simulink model "DCDC3_CL"  (R2024a)
settings: Solver=VariableStepAuto  StartTime=0.0  StopTime=Tsim_outLoop  FixedStep=Tstep  RelTol=1e-3
values from neighbouring files (symbols this model uses):
  deadtimesw = 2.8e-6    (= 2.8e-06)    [DCDC_param.m]
  ILmax = 3    [DCDC_param.m]
  Rload = VoutNom/IoutNom    (= 39.6825396825)    [DCDC_param.m]
  Tsw = 2.8e-6    (= 2.8e-06)    [DCDC_param.m]
  VinNom = 30    [DCDC_param.m]
  VoutNom = 50    [DCDC_param.m]
undefined symbols (not defined in the file or in its folder): den_aaf, DiscIntNeverNeededParam, kaw_i, kaw_v, ki_i, ki_v, kp_i, kp_v, kpf_i, kpf_v, num_aaf, Tstep, VLlim, zden_pf_i, zden_pf_v, znum_pf_i, znum_pf_v
libraries: simulink x30, nesl_utility x20, fl_lib x19, spsTriangleGeneratorLib x18, ee_lib x7
(part 1 of 2)
settings Model: Creator=nicholas  LastModifiedBy=nicholas
settings RTWCC: GPUComputeCapability=3.5

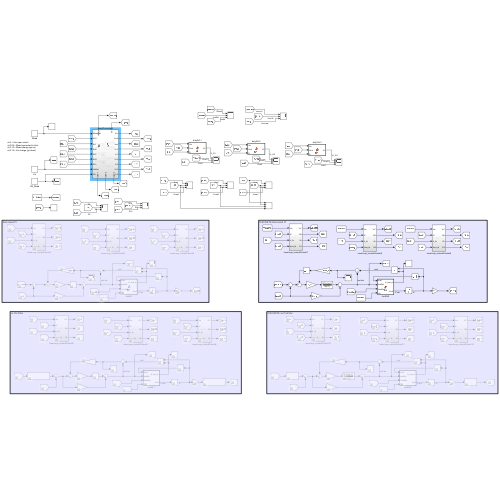
[thumbnail: Simulink's stored preview of the top-level diagram]
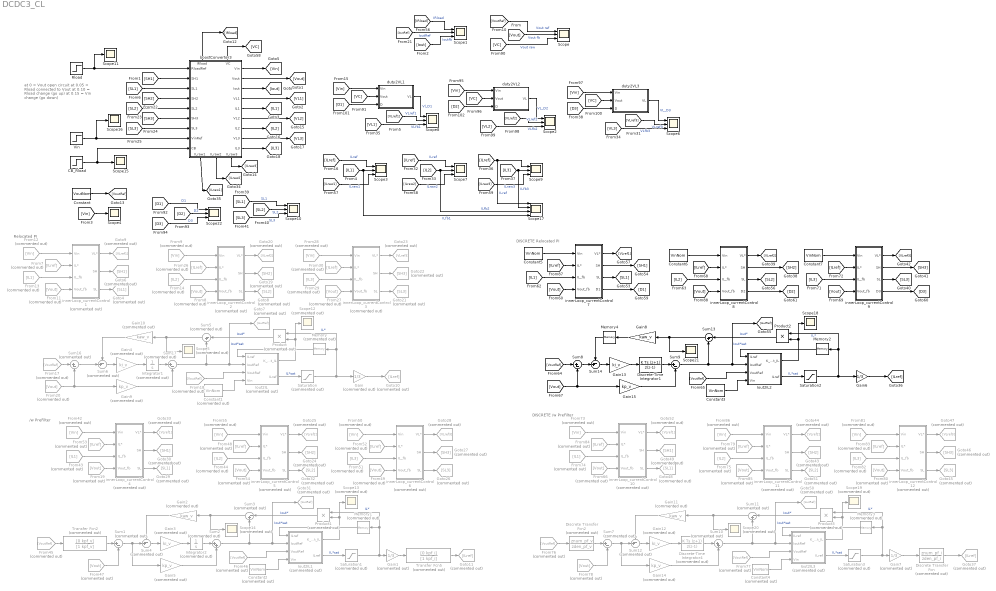
== system DCDC3_CL ==
  note: Relocated PI
  note: /w PreFilter
  note: at 0 = Vout open circuit
      | at 0.05 = Rload connected to Vout
      | at 0.10 = Rload change (go up)
      | at 0.15 = Vin change (go down)
  note: DISCRETE Relocated PI
  note: DISCRETE /w PreFilter
  CB_Rload : Step  Time=0.05  SampleTime=0
  Constant : Constant  Value=VoutNom
  Constant1 : Constant  Commented=on  Value=VinNom
  Constant2 : Constant  Commented=on  Value=VinNom
  Constant{3,5..7} (4 alike) : Constant  Value=VinNom
  Constant4 : Constant  Commented=on  Value=VinNom
  Discrete Transfer Fcn : DiscreteTransferFcn  Commented=on  Numerator=znum_pf_i  Denominator=zden_pf_i
  Discrete Transfer Fcn2 : DiscreteTransferFcn  Commented=on  Numerator=znum_pf_v  Denominator=zden_pf_v
  Discrete-Time Integrator1 : DiscreteIntegrator  IntegratorMethod=Integration: Trapezoidal  SampleTime=Tsw  ICPrevOutput=DiscIntNeverNeededParam  ICPrevScaledInput=DiscIntNeverNeededParam
  Discrete-Time Integrator4 : DiscreteIntegrator  Commented=on  IntegratorMethod=Integration: Trapezoidal  SampleTime=Tsw  ICPrevOutput=DiscIntNeverNeededParam  ICPrevScaledInput=DiscIntNeverNeededParam
  From{8,11,19..20,27,47,49,54,66,78,80,85} (12 alike) : From  Commented=on  GotoTag=Vout
  From{9,12,28,42,50,55,73,81,86} (9 alike) : From  Commented=on  GotoTag=Vin
  From13 : From  Commented=on  GotoTag=IL1
  From14 : From  Commented=on  GotoTag=IL2
  From{17..18,45..46,76..77} (6 alike) : From  Commented=on  GotoTag=VoutRef
  From{7,26,30,48,52..53,79,83..84} (9 alike) : From  Commented=on  GotoTag=ILref
  From29 : From  Commented=on  GotoTag=IL3
  From43 : From  Commented=on  GotoTag=IL1
  From44 : From  Commented=on  GotoTag=IL2
  From51 : From  Commented=on  GotoTag=IL3
  From74 : From  Commented=on  GotoTag=IL1
  From75 : From  Commented=on  GotoTag=IL2
  From82 : From  Commented=on  GotoTag=IL3
  Gain : Gain  Commented=on  Gain=1/3
  Gain1 : Gain  Commented=on  Gain=1/3
  Gain10 : Gain  Commented=on  Gain=kaw_v
  Gain11 : Gain  Commented=on  Gain=kaw_v
  Gain12 : Gain  Commented=on  Gain=ki_v
  Gain13 : Gain  Gain=ki_v
  Gain14 : Gain  Commented=on  Gain=kp_v
  Gain15 : Gain  Gain=kp_v
  Gain2 : Gain  Commented=on  Gain=kaw_v
  Gain3 : Gain  Commented=on  Gain=ki_v
  Gain4 : Gain  Commented=on  Gain=ki_v
  Gain5 : Gain  Commented=on  Gain=kp_v
  Gain6 : Gain  Gain=1/3
  Gain7 : Gain  Commented=on  Gain=1/3
  Gain8 : Gain  Gain=kaw_v
  Gain9 : Gain  Commented=on  Gain=kp_v
  Goto10 : Goto  Commented=on  GotoTag=ILref
  Goto11 : Goto  Commented=on  GotoTag=ILref
  Goto19 : Goto  Commented=on  GotoTag=SH2
  Goto20 : Goto  Commented=on  GotoTag=VLref2
  Goto21 : Goto  Commented=on  GotoTag=SL3
  Goto22 : Goto  Commented=on  GotoTag=SH3
  Goto23 : Goto  Commented=on  GotoTag=VLref3
  Goto24 : Goto  Commented=on  GotoTag=SH2
  Goto25 : Goto  Commented=on  GotoTag=VLref2
  Goto26 : Goto  Commented=on  GotoTag=SL3
  Goto27 : Goto  Commented=on  GotoTag=SH3
  Goto28 : Goto  Commented=on  GotoTag=VLref3
  Goto29 : Goto  Commented=on  GotoTag=SL1
  Goto30 : Goto  Commented=on  GotoTag=SH1
  Goto31 : Goto  Commented=on  GotoTag=IoutRef
  Goto32 : Goto  Commented=on  GotoTag=SL2
  Goto33 : Goto  Commented=on  GotoTag=VLref1
  Goto37 : Goto  Commented=on  GotoTag=ILref
  Goto4 : Goto  Commented=on  GotoTag=SL1
  Goto43 : Goto  Commented=on  GotoTag=SH2
  Goto44 : Goto  Commented=on  GotoTag=VLref2
  Goto45 : Goto  Commented=on  GotoTag=SL3
  Goto46 : Goto  Commented=on  GotoTag=SH3
  Goto47 : Goto  Commented=on  GotoTag=VLref3
  Goto48 : Goto  Commented=on  GotoTag=SL1
  Goto49 : Goto  Commented=on  GotoTag=SH1
  Goto50 : Goto  Commented=on  GotoTag=IoutRef
  Goto51 : Goto  Commented=on  GotoTag=SL2
  Goto52 : Goto  Commented=on  GotoTag=VLref1
  Goto6 : Goto  Commented=on  GotoTag=SH1
  Goto7 : Goto  Commented=on  GotoTag=IoutRef
  Goto8 : Goto  Commented=on  GotoTag=SL2
  Goto9 : Goto  Commented=on  GotoTag=VLref1
  Integrator1 : Integrator  Commented=on
  Integrator2 : Integrator  Commented=on
  Iout2IL : MATLAB Function  Commented=on  TreatAsAtomicUnit=on
  Iout2IL1 : MATLAB Function  Commented=on  TreatAsAtomicUnit=on
  Iout2IL2 : MATLAB Function  TreatAsAtomicUnit=on
  Iout2IL3 : MATLAB Function  Commented=on  TreatAsAtomicUnit=on
  Memory : Memory  Commented=on
  Memory1 : Memory  Commented=on
  Memory2 : Memory
  Memory3 : Memory  Commented=on
  Memory4 : Memory
  Product : Product  Commented=on
  Product1 : Product  Commented=on
  Product2 : Product
  Product3 : Product  Commented=on
  Rload : Step  Time=0.1  Before=Rload  After=Rload*2  SampleTime=0
  Saturation : Saturate  Commented=on  UpperLimit=ILmax  LowerLimit=-ILmax
  Saturation1 : Saturate  Commented=on  UpperLimit=ILmax  LowerLimit=-ILmax
  Saturation2 : Saturate  UpperLimit=ILmax  LowerLimit=-ILmax
  Saturation3 : Saturate  Commented=on  UpperLimit=ILmax  LowerLimit=-ILmax
  Scope{,1..3,6..10,22} (10 alike) : Scope  NumInputPorts=3
  Scope{4,11,15..16,18,21} (6 alike) : Scope
  Scope{5,12..14,19..20} (6 alike) : Scope  Commented=on
  Scope17 : Scope  NumInputPorts=4
  Sum{1,7,16..17} (4 alike) : Sum  Commented=on  Inputs=|+-
  Sum10 : Sum  Commented=on  Inputs=|++
  Sum11 : Sum  Commented=on  Inputs=|-+
  Sum12 : Sum  Commented=on  Inputs=-+|
  Sum13 : Sum  Inputs=|-+
  Sum14 : Sum  Inputs=-+|
  Sum2 : Sum  Commented=on  Inputs=|++
  Sum3 : Sum  Commented=on  Inputs=|-+
  Sum4 : Sum  Commented=on  Inputs=-+|
  Sum5 : Sum  Commented=on  Inputs=|-+
  Sum6 : Sum  Commented=on  Inputs=-+|
  Sum8 : Sum  Inputs=|+-
  Sum9 : Sum  Inputs=|+-
  Transfer Fcn2 : TransferFcn  Commented=on  Numerator=[0 kpf_v]  Denominator=[1 kpf_v]
  Transfer Fcn5 : TransferFcn  Commented=on  Numerator=[0 kpf_i]  Denominator=[1 kpf_i]
  Vin : Step  Time=0.15  Before=VinNom  After=20  SampleTime=0
  boostConverter3 : Subsystem
      settings: PortSchema="{\"entries\":[{\"content\":{\"sides\":[{\"content\":{\"connectorIds\":[\"In1\",\"In2\",\"In3\",\"In4\",\"In5\",\"In6\",\"In7\",\"In8\",\"In9\"]},\"type\":\"ConnectorPlacement.EquallySpacedRectSide\",\"uuid\":\"b55511d0-facb-4a91-89ed-441d6ed333ad\"},{\"content\":{\"connectorIds\":[\"Out1\",\"Out2\",\"Out3\",\"Out4\",\"Out5\",\"Out6\",\"Out7\",\"Out8\",\"Out9\"],\"side\":\"RIGHT\"},\"type\":\"ConnectorPlacement.EquallySpacedRectSide\",\"uuid\":\"ead4c989-543f-44ce-a846-94a06a8e7cad\"},{\"content\":{\"connectorIds\":[\"Out13\",\"Out14\"],\"side\":\"TOP\"},\"type\":\"ConnectorPlacement.EquallySpacedRectSide\",\"uuid\":\"5dda5bdb-be03-4339-a562-891a6c50bbdd\"},{\"content\":{\"connectorIds\":[\"Out10\",\"Out11\",\"Out12\"],\"side\":\"BOTTOM\"},\"type\":\"ConnectorPlacement.EquallySpacedRectSide\",\"uuid\":\"6ce891dd-de23-45e8-b9d4-5962e703d661\"}]},\"type\":\"ConnectorPlacement.EquallySpacedConnector\",\"uuid\":\"250b2e18-3b96-4cfc-be30-976dd92f9027\"}],\"packageUris\":[\"http://schema.mathworks.com/mf0/Connector/R2020b\"],\"version\":\"1.0\"}"
  duty2VL1 : MATLAB Function  TreatAsAtomicUnit=on
  duty2VL2 : MATLAB Function  TreatAsAtomicUnit=on
  duty2VL3 : MATLAB Function  TreatAsAtomicUnit=on
  innerLoop_currentControl1 : Subsystem  Commented=on
  innerLoop_currentControl10 : Subsystem  Commented=on
  innerLoop_currentControl11 : Subsystem  Commented=on
  innerLoop_currentControl12 : Subsystem  Commented=on
  innerLoop_currentControl2 : Subsystem  Commented=on
  innerLoop_currentControl3 : Subsystem  Commented=on
  innerLoop_currentControl4 : Subsystem  Commented=on
  innerLoop_currentControl5 : Subsystem  Commented=on
  innerLoop_currentControl6 : Subsystem  Commented=on
  innerLoop_currentControl7 : Subsystem
  innerLoop_currentControl8 : Subsystem
  innerLoop_currentControl9 : Subsystem
  wires:
  [Iout] -> Scope1/3  "Ioutfb"
  [IL1] -> Scope17/4, Scope3/2  "ILfb1"
  boostConverter3/3(Iout) -> [Iout]
  boostConverter3/2(Vout) -> [Vout]
  boostConverter3/4(VL1) -> [VL1]
  boostConverter3/5(IL1) -> [IL1]
  boostConverter3/1(Vin) -> [Vin]
  [SL1] -> boostConverter3/3(SL1)
  [SH1] -> boostConverter3/2(SH1)
  [ILref] -> Scope3/1  "ILref"
  [IoutRef] -> Scope1/2  "IoutRef"
  Constant/1 -> [VoutRef]
  boostConverter3/6(VL2) -> [VL2]
  boostConverter3/7(IL2) -> [IL2]
  boostConverter3/8(VL3) -> [VL3]
  boostConverter3/9(IL3) -> [IL3]
  [SL2] -> boostConverter3/5(SL2)
  [SH2] -> boostConverter3/4(SH2)
  [SL3] -> boostConverter3/7(SL3)
  [SH3] -> boostConverter3/6(SH3)
  From12/1 -> innerLoop_currentControl1/1(Vin)
  From7/1 -> innerLoop_currentControl1/2(IL*)
  From13/1 -> innerLoop_currentControl1/3(IL_fb)
  From11/1 -> innerLoop_currentControl1/4(Vout_fb)
  innerLoop_currentControl1/1(VL*) -> Goto9/1
  innerLoop_currentControl1/2(SH) -> Goto6/1
  innerLoop_currentControl1/3(SL) -> Goto4/1
  From9/1 -> innerLoop_currentControl2/1(Vin)
  innerLoop_currentControl2/1(VL*) -> Goto20/1
  From26/1 -> innerLoop_currentControl2/2(IL*)
  innerLoop_currentControl2/3(SL) -> Goto8/1
  From14/1 -> innerLoop_currentControl2/3(IL_fb)
  From8/1 -> innerLoop_currentControl2/4(Vout_fb)
  innerLoop_currentControl2/2(SH) -> Goto19/1
  From28/1 -> innerLoop_currentControl3/1(Vin)
  innerLoop_currentControl3/1(VL*) -> Goto23/1
  From30/1 -> innerLoop_currentControl3/2(IL*)
  innerLoop_currentControl3/3(SL) -> Goto21/1
  From29/1 -> innerLoop_currentControl3/3(IL_fb)
  From27/1 -> innerLoop_currentControl3/4(Vout_fb)
  innerLoop_currentControl3/2(SH) -> Goto22/1
  [IL2] -> Scope7/2, Scope17/3  "ILfb2"
  [ILref] -> Scope7/1  "ILref"
  [IL3] -> Scope17/2, Scope9/2  "ILfb3"
  [ILref] -> Scope17/1, Scope9/1  "ILref"
  [SL1] -> Scope10/1  "SL1"
  [SL2] -> Scope10/2  "SL2"
  [SL3] -> Scope10/3  "SL3"
  From20/1 -> Gain9/1, Sum16/2
  Integrator1/1 -> Sum17/1
  Iout2IL/2(ILref) -> Saturation/1  "IL*sat"
  Saturation/1 -> Product/1, Memory/1, Gain/1  "IL*"
  From17/1 -> Sum16/1
  Sum17/1 -> Sum5/2, Iout2IL/2(IoutRef), Goto7/1  "Iout*sat"
  Gain4/1 -> Integrator1/1
  Sum5/1 -> Scope5/1, Gain10/1
  Memory/1 -> Iout2IL/1("ILref ")
  Gain9/1 -> Sum17/2
  Gain10/1 -> Sum6/1
  Sum16/1 -> Sum6/2
  Product/1 -> Sum5/1  "Iout*"
  Iout2IL/1(K_Iout_IL) -> Product/2, Scope12/1
  Sum6/1 -> Gain4/1
  Constant1/1 -> Iout2IL/4(Vin)
  From18/1 -> Iout2IL/3(VoutRef)
  Gain/1 -> Goto10/1
  Constant2/1 -> Iout2IL1/4(Vin)
  Sum4/1 -> Gain3/1
  From46/1 -> Iout2IL1/3(VoutRef)
  Sum1/1 -> Gain5/1, Sum4/2
  Sum3/1 -> Scope14/1, Gain2/1
  Memory1/1 -> Iout2IL1/1("ILref ")
  Integrator2/1 -> Sum2/1
  From45/1 -> Transfer Fcn2/1
  Saturation1/1 -> Product1/1, Memory1/1, Gain1/1  "IL*"
  From47/1 -> Sum1/2
  Iout2IL1/1(K_Iout_IL) -> Product1/2, Scope13/1
  Product1/1 -> Sum3/1  "Iout*"
  Gain2/1 -> Sum4/1
  From51/1 -> innerLoop_currentControl6/3(IL_fb)
  From44/1 -> innerLoop_currentControl5/3(IL_fb)
  From52/1 -> innerLoop_currentControl6/2(IL*)
  From55/1 -> innerLoop_currentControl5/1(Vin)
  Sum2/1 -> Sum3/2, Iout2IL1/2(IoutRef), Goto31/1  "Iout*sat"
  innerLoop_currentControl5/3(SL) -> Goto32/1
  From43/1 -> innerLoop_currentControl4/3(IL_fb)
  From53/1 -> innerLoop_currentControl4/2(IL*)
  From54/1 -> innerLoop_currentControl5/4(Vout_fb)
  innerLoop_currentControl4/2(SH) -> Goto30/1
  innerLoop_currentControl6/2(SH) -> Goto27/1
  From19/1 -> innerLoop_currentControl4/4(Vout_fb)
  Gain5/1 -> Sum2/2
  innerLoop_currentControl4/1(VL*) -> Goto33/1
  From42/1 -> innerLoop_currentControl4/1(Vin)
  From50/1 -> innerLoop_currentControl6/1(Vin)
  innerLoop_currentControl5/2(SH) -> Goto24/1
  Gain3/1 -> Integrator2/1
  innerLoop_currentControl5/1(VL*) -> Goto25/1
  From48/1 -> innerLoop_currentControl5/2(IL*)
  innerLoop_currentControl6/3(SL) -> Goto26/1
  innerLoop_currentControl4/3(SL) -> Goto29/1
  innerLoop_currentControl6/1(VL*) -> Goto28/1
  From49/1 -> innerLoop_currentControl6/4(Vout_fb)
  Gain1/1 -> Transfer Fcn5/1
  Iout2IL1/2(ILref) -> Saturation1/1  "IL*sat"
  Transfer Fcn2/1 -> Sum1/1
  Transfer Fcn5/1 -> Goto11/1
  Vin/1 -> Scope16/1, boostConverter3/8(VinRef)
  Rload/1 -> boostConverter3/1(RloadRef), Scope11/1
  CB_Rload/1 -> boostConverter3/9(CB), Scope15/1
  boostConverter3/13(IRload) -> [IRload]
  [IRload] -> Scope1/1  "IRload"
  boostConverter3/12(ILraw3) -> [ILraw3]
  boostConverter3/11(ILraw2) -> [ILraw2]
  boostConverter3/10(ILraw1) -> [ILraw1]
  [ILraw1] -> Scope3/3  "ILraw1"
  [ILraw2] -> Scope7/3  "ILraw2"
  [ILraw3] -> Scope9/3  "ILraw3"
  Sum13/1 -> Scope21/1, Gain8/1
  innerLoop_currentControl8/3(SL) -> [SL2]
  From66/1 -> innerLoop_currentControl10/4(Vout_fb)
  Discrete-Time Integrator4/1 -> Sum10/1
  From73/1 -> innerLoop_currentControl10/1(Vin)
  innerLoop_currentControl10/3(SL) -> Goto48/1
  Sum14/1 -> Gain13/1
  Discrete Transfer Fcn2/1 -> Sum7/1
  Product2/1 -> Sum13/1  "Iout*"
  Discrete Transfer Fcn/1 -> Goto37/1
  Gain7/1 -> Discrete Transfer Fcn/1
  From75/1 -> innerLoop_currentControl11/3(IL_fb)
  From80/1 -> innerLoop_currentControl12/4(Vout_fb)
  innerLoop_currentControl11/2(SH) -> Goto43/1
  [VoutRef] -> Sum8/1
  innerLoop_currentControl12/1(VL*) -> Goto47/1
  innerLoop_currentControl11/3(SL) -> Goto51/1
  Gain14/1 -> Sum10/2
  Constant6/1 -> innerLoop_currentControl8/1(Vin)
  Iout2IL3/2(ILref) -> Saturation3/1  "IL*sat"
  innerLoop_currentControl12/3(SL) -> Goto45/1
  Sum10/1 -> Sum11/2, Iout2IL3/2(IoutRef), Goto50/1  "Iout*sat"
  Sum8/1 -> Sum14/2
  [Vout] -> Gain15/1, Sum8/2
  Gain6/1 -> [ILref]
  From74/1 -> innerLoop_currentControl10/3(IL_fb)
  innerLoop_currentControl12/2(SH) -> Goto46/1
  Gain12/1 -> Discrete-Time Integrator4/1
  innerLoop_currentControl11/1(VL*) -> Goto44/1
  innerLoop_currentControl9/3(SL) -> [SL3]
  From82/1 -> innerLoop_currentControl12/3(IL_fb)
  Memory3/1 -> Iout2IL3/1("ILref ")
  From81/1 -> innerLoop_currentControl12/1(Vin)
  From85/1 -> innerLoop_currentControl11/4(Vout_fb)
  innerLoop_currentControl10/2(SH) -> Goto49/1
  Gain8/1 -> Memory4/1
  innerLoop_currentControl7/1(VL*) -> [VLref1]
  From84/1 -> innerLoop_currentControl10/2(IL*)
  From76/1 -> Discrete Transfer Fcn2/1
  Iout2IL2/1(K_Iout_IL) -> Product2/2, Scope18/1
  Gain11/1 -> Sum12/1
  From83/1 -> innerLoop_currentControl12/2(IL*)
  Iout2IL3/1(K_Iout_IL) -> Product3/2, Scope19/1
  Product3/1 -> Sum11/1  "Iout*"
  From78/1 -> Sum7/2
  innerLoop_currentControl8/2(SH) -> [SH2]
  Saturation3/1 -> Product3/1, Memory3/1, Gain7/1  "IL*"
  Sum11/1 -> Scope20/1, Gain11/1
  [VoutRef] -> Iout2IL2/3(VoutRef)
  Sum12/1 -> Gain12/1
  Memory2/1 -> Iout2IL2/1("ILref ")
  Constant3/1 -> Iout2IL2/4(Vin)
  From77/1 -> Iout2IL3/3(VoutRef)
  Constant4/1 -> Iout2IL3/4(Vin)
  [ILref] -> innerLoop_currentControl8/2(IL*)
  [IL3] -> innerLoop_currentControl9/3(IL_fb)
  [Vout] -> innerLoop_currentControl7/4(Vout_fb)
  Saturation2/1 -> Product2/1, Memory2/1, Gain6/1  "IL*"
  Sum9/1 -> Sum13/2, Iout2IL2/2(IoutRef), [IoutRef]  "Iout*sat"
  [IL2] -> innerLoop_currentControl8/3(IL_fb)
  innerLoop_currentControl10/1(VL*) -> Goto52/1
  Discrete-Time Integrator1/1 -> Sum9/1
  Iout2IL2/2(ILref) -> Saturation2/1  "IL*sat"
  Gain13/1 -> Discrete-Time Integrator1/1
  From86/1 -> innerLoop_currentControl11/1(Vin)
  [ILref] -> innerLoop_currentControl9/2(IL*)
  Sum7/1 -> Gain14/1, Sum12/2
  Constant7/1 -> innerLoop_currentControl9/1(Vin)
  [Vout] -> innerLoop_currentControl8/4(Vout_fb)
  [Vout] -> innerLoop_currentControl9/4(Vout_fb)
  innerLoop_currentControl9/2(SH) -> [SH3]
  Constant5/1 -> innerLoop_currentControl7/1(Vin)
  innerLoop_currentControl8/1(VL*) -> [VLref2]
  [ILref] -> innerLoop_currentControl7/2(IL*)
  innerLoop_currentControl7/3(SL) -> [SL1]
  From79/1 -> innerLoop_currentControl11/2(IL*)
  innerLoop_currentControl9/1(VL*) -> [VLref3]
  [IL1] -> innerLoop_currentControl7/3(IL_fb)
  innerLoop_currentControl7/2(SH) -> [SH1]
  Gain15/1 -> Sum9/2
  [VoutRef] -> Scope/1  "Vout ref"
  [Vout] -> Scope/2  "Vout fb"
  [VC] -> Scope/3  "Vout raw"
  boostConverter3/14(VC) -> [VC]
  [D3] -> Scope22/3  "D3"
  [D1] -> Scope22/1  "D1"
  [D2] -> Scope22/2  "D2"
  innerLoop_currentControl8/4(D2) -> [D2]
  innerLoop_currentControl7/4(D1) -> [D1]
  innerLoop_currentControl9/4(D3) -> [D3]
  [Vin] -> Scope4/1
  [VL1] -> Scope8/3  "VLfb1"
  [VLref1] -> Scope8/2  "VLref1"
  [VL3] -> Scope6/3  "VLfb3"
  [VLref3] -> Scope6/2  "VLref3"
  [D1] -> duty2VL1/3(D)
  duty2VL2/1(VL) -> Scope2/1  "VL_D2"
  duty2VL3/1(VL) -> Scope6/1  "VL_D3"
  [Vin] -> duty2VL2/1(Vin)
  [VC] -> duty2VL2/2(Vout)
  [VC] -> duty2VL1/2(Vout)
  [Vin] -> duty2VL1/1(Vin)
  [Vin] -> duty2VL3/1(Vin)
  duty2VL1/1(VL) -> Scope8/1  "Vl_D1"
  [D2] -> duty2VL2/3(D)
  [VLref2] -> Scope2/2  "VLref2"
  [VC] -> duty2VL3/2(Vout)
  [D3] -> duty2VL3/3(D)
  [VL2] -> Scope2/3  "VLfb2"
  Memory4/1 -> Sum14/1

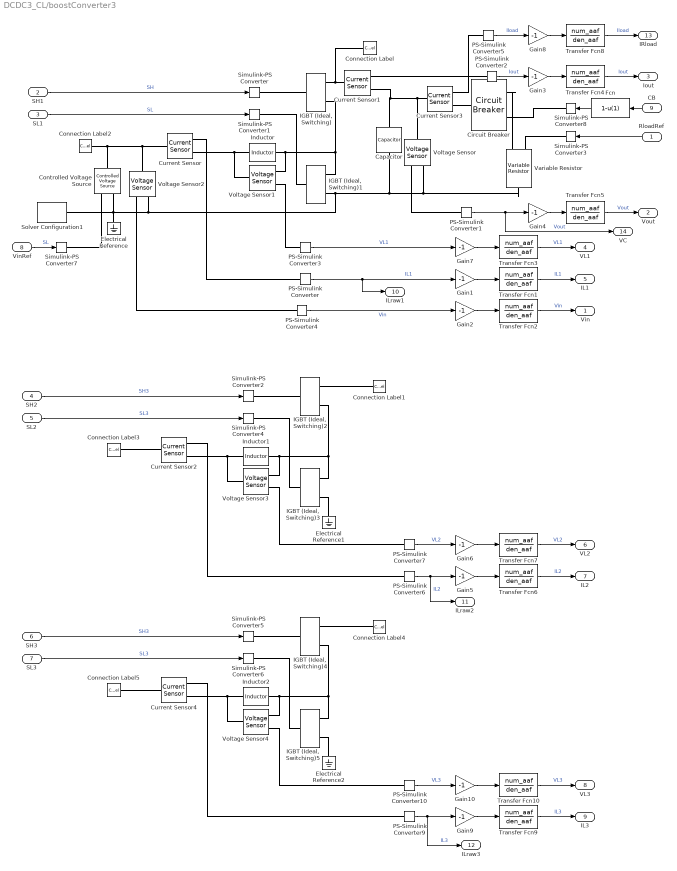
== system DCDC3_CL/boostConverter3 ==
  RloadRef : Inport
  SH1 : Inport  Port=2
  SL1 : Inport  Port=3
  SH2 : Inport  Port=4
  SL2 : Inport  Port=5
  SH3 : Inport  Port=6
  SL3 : Inport  Port=7
  VinRef : Inport  Port=8
  CB : Inport  Port=9
  Capacitor : fl_lib/Electrical/Electrical Elements/Capacitor  c=C F  r=RserC Ohm  g=0 1/Ohm  i_specify=off  i_priority=None  i=0 A  i_nominal_specify=off  i_nominal_value=1  i_nominal_unit=A  v_specify=off  v_priority=High  v=VoutNom V  v_nominal_specify=off  v_nominal_value=1  v_nominal_unit=V  vc_specify=off  vc_priority=High  vc=0 V  vc_nominal_specify=off  vc_nominal_value=1  vc_nominal_unit=V
  Circuit Breaker : ee_lib/Switches & Breakers/Circuit Breaker  R_closed=1e-9 Ohm  G_open=1e-9 1/Ohm  threshold=0.5 V  breaker_behavior=ee.enum.switches.breakerBehavior.zeroCrossingDisable
      settings: InternalSimscapePortConfiguration="{\"Bottom\":[],\"Left\":[{\"id\":\"vT\",\"label\":\"vT\",\"type\":\"input\"},{\"id\":\"p1\",\"label\":\"\",\"type\":\"foundation.electrical.electrical\"}],\"Right\":[{\"id\":\"p2\",\"label\":\"\",\"type\":\"foundation.electrical.electrical\"}],\"Top\":[]}"
  Connection Label : ConnectionLabel  Label=Vout_DClink
  Connection Label1 : ConnectionLabel  Label=Vout_DClink
  Connection Label2 : ConnectionLabel  Label=Vin
  Connection Label3 : ConnectionLabel  Label=Vin
  Connection Label4 : ConnectionLabel  Label=Vout_DClink
  Connection Label5 : ConnectionLabel  Label=Vin
  Controlled Voltage Source : fl_lib/Electrical/Electrical Sources/Controlled Voltage Source
  Current Sensor{,1..4} (5 alike) : fl_lib/Electrical/Electrical Sensors/Current Sensor
  Electrical Reference : fl_lib/Electrical/Electrical Elements/Electrical Reference
  Electrical Reference1 : fl_lib/Electrical/Electrical Elements/Electrical Reference
  Electrical Reference2 : fl_lib/Electrical/Electrical Elements/Electrical Reference
  Fcn : Fcn  Expr=1-u(1)
  Gain{1..10} (10 alike) : Gain  Gain=-1
  IGBT (Ideal, Switching){,1..5} (6 alike) : ee_lib/Semiconductors & Converters/IGBT (Ideal, Switching)  port_option=ee.enum.controlport.ps  Vf=0.8 V  Ron=0.001 Ohm  Goff=1e-5 1/Ohm  Vth=VthIGBT V  diode_param=ee.enum.converters.protectiondiode.nodynamics  diode_Vf=0.8 V  diode_Ron=0.001 Ohm  diode_Goff=1e-5 1/Ohm  diode_C=50e-9 F  diode_iRM=-235 A  diode_iF=300 A  diode_idot=-50 A/us  diode_trr_param=ee.enum.converters.diodeReverseParam.trr_factor  diode_trr_factor=3  diode_trr=15 us  diode_Qrr=1500 s*uA  ice_specify=off  ice_priority=None  ice=0 A  ice_nominal_specify=off  ice_nominal_value=1  ice_nominal_unit=A  vce_specify=off  vce_priority=None  vce=0 V  vce_nominal_specify=off  vce_nominal_value=1  vce_nominal_unit=V  vge_specify=off  vge_priority=None  vge=0 V  vge_nominal_specify=off  vge_nominal_value=1  vge_nominal_unit=V  thermal_loss_option=ee.enum.converters.thermalLossOption.constantvalues  Von_data=[0, .1, .6, .8, 1, 1.3, 1.6, 2, 2.4; 0, .1, .7, 1, 1.2, 1.5, 1.9, 2.4, 2.8] V  Tj=[298.15, 398.15] K  Iout_data=[0, .1, 1, 5, 10, 20, 40, 70, 100] A  Eon_data=[0, .0024, .024, .12, .2, .48, 1.04, 2.16, 3.24; 0, .003, .03, .15, .25, .6, 1.3, 2.7, 4.05] * 1e-3 J  Eoff_data=[0, .0007, .0066, .033, .066, .17, .33, .83, 1.5; 0, .001, .01, .05, .1, .25, .5, 1.2, 2.2] * 1e-3 J  Eon_data_3D=[zeros(2, 9, 3)] J  Eoff_data_3D=[zeros(2, 9, 3)] J  Tj_loss=[298.15, 398.15] K  Iout_data_loss=[0, .1, 1, 5, 10, 20, 40, 70, 100] A  tabulateWithVce=false  Vce_loss=[0, 150, 300] V  Eon_scalar=22.86e-3 J  Eoff_scalar=17.14e-3 J  Voff=300 V  Iout_scalar=600 A  useCurrentFromPreviousCycle=false  useVoltageFromPreviousCycle=false  diodeModelType=ee.enum.converters.diodeModelType.pwl  diodeTableType=ee.enum.diode.tableType.IfMat  diode_ReverseIVType=ee.enum.diode.diodeReverseIV.constant  diode_IfMat=[.07, .12, .19, 1.75, 4.24, 7.32, 11.2; .16, .3, .72, 2.14, 4.02, 6.35, 9.12] A  diode_VfMat=[.9, 1.15, 1.25, 1.5, 1.75, 2.17, 2.6, 2.85; .58, .68, .75, 1.1, 1.38, 1.77, 2.27, 2.7] V  diode_TjVec=[25, 125] degC  diode_VfVec=[.5, .7, .9, 1.3, 1.7, 2.1, 2.5] V  diode_IfVec=[.1, .2, .5, 1, 2, 4, 7, 10] A  diode_IrMat=[1e-06, 2e-06, 5e-06, 1e-05, 2.5e-05, 5e-05, .0001; 2e-06, 5e-06, 1e-05, 4e-05, 8e-05, .0002, .0005] A  diode_VrMat=[10, 100, 200, 250, 300, 325, 350; 10, 70, 160, 220, 270, 300, 320] V  diode_VrVec=[10, 20, 40, 50, 70, 80, 100] V  diode_IrVec=[1e-06, 2e-06, 5e-06, 1e-05, 2e-05, 5e-05, .0001] A  diode_Vr=-600 V  diode_Ls=150 nH  diode_Erec=0.03 J  diode_rec_loss_model=ee.enum.diode.reverseRecoveryModel.fixed  diode_ErecVal=0 J  diode_scaleWithIandV=true  diode_ErecMat=zeros(2, 3) J  diode_TjrecVec=[298.15, 398.15] K  diode_IfrecVec=[.1, 1, 10] A  diode_IrecVal=10 A  diode_VrecVal=10 V  diode_tFilter=1 / 1000 / 100 s  thermal_network_parameterization=ee.enum.thermalNetworkTopology.external  Rth=[.08, .5] K/W  Rth_Cauer=[.08, .1, .5] K/W  Rth_Foster=[.08, .14, .22, .16] K/W  thermal_mass_parameterization=ee.enum.thermalNetwork.timeconstant  thermal_mass=[.01, .5] J/K  thermal_mass_Cauer=[.01, .1, .5] J/K  thermal_mass_Foster=[.001, .005, .05, .5] J/K  thermal_time_constant=[.001, .2] s  thermal_time_constant_Cauer=[.001, .1, .2] s  thermal_time_constant_Foster=[7e-05, .0007, .01, .08] s  thermal_mass_initial_temperatures=[25, 25] degC  thermal_mass_initial_temperatures_Cauer=[25, 25, 25] degC  junction_thermal_mass=0.01 J/K  Tvec_initial_Foster=[25, 25, 25, 25] degC  no_thermal_network=0  junction_temperature_specify=off  junction_temperature_priority=None  junction_temperature=25 degC  junction_temperature_nominal_specify=off  junction_temperature_nominal_value=1  junction_temperature_nominal_unit=degC  Qj_specify=off  Qj_priority=None  Qj=0 W  Qj_nominal_specify=off  Qj_nominal_value=1  Qj_nominal_unit=W  accumulatedSwitchingLosses_specify=off  accumulatedSwitchingLosses_priority=None  accumulatedSwitchingLosses=0 J
  Inductor : fl_lib/Electrical/Electrical Elements/Inductor  l=L H  r=RserL Ohm  g=1e-9 1/Ohm  i_specify=off  i_priority=None  i=Iin A  i_nominal_specify=off  i_nominal_value=1  i_nominal_unit=A  v_specify=off  v_priority=None  v=0 V  v_nominal_specify=off  v_nominal_value=1  v_nominal_unit=V  i_L_specify=off  i_L_priority=High  i_L=0 A  i_L_nominal_specify=off  i_L_nominal_value=1  i_L_nominal_unit=A
  Inductor1 : fl_lib/Electrical/Electrical Elements/Inductor  l=L H  r=RserL Ohm  g=1e-9 1/Ohm  i_specify=off  i_priority=None  i=Iin A  i_nominal_specify=off  i_nominal_value=1  i_nominal_unit=A  v_specify=off  v_priority=None  v=0 V  v_nominal_specify=off  v_nominal_value=1  v_nominal_unit=V  i_L_specify=off  i_L_priority=High  i_L=0 A  i_L_nominal_specify=off  i_L_nominal_value=1  i_L_nominal_unit=A
  Inductor2 : fl_lib/Electrical/Electrical Elements/Inductor  l=L H  r=RserL Ohm  g=1e-9 1/Ohm  i_specify=off  i_priority=None  i=Iin A  i_nominal_specify=off  i_nominal_value=1  i_nominal_unit=A  v_specify=off  v_priority=None  v=0 V  v_nominal_specify=off  v_nominal_value=1  v_nominal_unit=V  i_L_specify=off  i_L_priority=High  i_L=0 A  i_L_nominal_specify=off  i_L_nominal_value=1  i_L_nominal_unit=A
  PS-Simulink Converter{,1..7,9..10} (10 alike) : nesl_utility/PS-Simulink Converter  PhysicalDomain=network_engine_domain  SubClassName=ps_output  LeftPortType=input  RightPortType=output  PseudoPeriodic=off  Frequencies=[]  VectorFormat=inherit  Unit=inherit  AffineConversion=off
  Simulink-PS Converter{,1..2,4..6,8} (7 alike) : nesl_utility/Simulink-PS Converter  PhysicalDomain=network_engine_domain  SubClassName=ps_input  LeftPortType=input  RightPortType=output  PseudoPeriodic=off  Frequencies=[]  NoiseDistribution=none  NoiseParameters=[]  Unit=1  AffineConversion=off  FilteringAndDerivatives=provide  SimscapeFilterOrder=1  InputFilterTimeConstant=0.001  UdotUserProvided=0
  Simulink-PS Converter3 : nesl_utility/Simulink-PS Converter  PhysicalDomain=network_engine_domain  SubClassName=ps_input  LeftPortType=input  RightPortType=output  PseudoPeriodic=off  Frequencies=[]  NoiseDistribution=none  NoiseParameters=[]  Unit=1  AffineConversion=off  FilteringAndDerivatives=filter  SimscapeFilterOrder=1  InputFilterTimeConstant=Tstep  UdotUserProvided=0
  Simulink-PS Converter7 : nesl_utility/Simulink-PS Converter  PhysicalDomain=network_engine_domain  SubClassName=ps_input  LeftPortType=input  RightPortType=output  PseudoPeriodic=off  Frequencies=[]  NoiseDistribution=none  NoiseParameters=[]  Unit=1  AffineConversion=off  FilteringAndDerivatives=filter  SimscapeFilterOrder=1  InputFilterTimeConstant=Tstep  UdotUserProvided=0
  Solver Configuration1 : nesl_utility/Solver Configuration  PhysicalDomain=network_engine_domain  SubClassName=solver  LeftPortType=input  RightPortType=generic  Tones=[]  Harmonics=[]  SimulateNoise=off  Profile=off  UseLocalSampling=off  EnableSwitchedLinearOptims=on  FrequencyDomain=off  UseCCode=off  RelTol=0.001  AbsTol=1e-06  MinStep=1e-09  ToWorkspace=off  RevertToSquareIcSolve=off  NumHomotopyIterations=100  PhasorMode=off  PhasorModeNumHarmonics=1  ConsistencySolver=NEWTON_FTOL  IndexReductionMethod=DerivativeReplacement  DoDC=off  ResidualTolerance=1e-09  ConsistencyTolSource=GLOBAL  ConsistencyAbsTol=0.001  ConsistencyRelTol=0.001  ConsistencyTolFactor=0.001  UseLocalSolver=off  LocalSolverChoice=NE_TRAPEZOIDAL_ADVANCER  ResolveIndetEquations=on  FunctionEvalNumThread=1  LocalSolverSampleTime=Tstep  DoFixedCost=off  MaxNonlinIter=3  MaxModeIter=2  ComputeImpulses=off  ImpulseIterations=2  LinearAlgebra=auto  LinearAlgebraNumThread=0  EquationFormulation=NE_TIME_EF  DelaysMemoryBudget=1024  AutomaticFiltering=off  FilteringTimeConstant=0.001  PartitionStorageMethod=AS_NEEDED  PartitionMemoryBudget=1024  PartitionMethod=ROBUST  MultibodyUseLocalSolver=off  MultibodyLocalSolverChoice=ODE1  MultibodyLocalSolverSampleTime=0.001
  Transfer Fcn{1..10} (10 alike) : TransferFcn  Numerator=num_aaf  Denominator=den_aaf
  Variable Resistor : fl_lib/Electrical/Electrical Elements/Variable Resistor  Rmin=Rload*0.9 Ohm  thermalEnable=false  thermal_mass=1 J/K  i_specify=off  i_priority=None  i=0 A  i_nominal_specify=off  i_nominal_value=1  i_nominal_unit=A  v_specify=off  v_priority=None  v=0 V  v_nominal_specify=off  v_nominal_value=1  v_nominal_unit=V  T_specify=off  T_priority=None  T=300 K  T_nominal_specify=off  T_nominal_value=1  T_nominal_unit=K
  Voltage Sensor{,1..4} (5 alike) : fl_lib/Electrical/Electrical Sensors/Voltage Sensor
  Vin : Outport
  Vout : Outport  Port=2
  Iout : Outport  Port=3
  VL1 : Outport  Port=4
  IL1 : Outport  Port=5
  VL2 : Outport  Port=6
  IL2 : Outport  Port=7
  VL3 : Outport  Port=8
  IL3 : Outport  Port=9
  ILraw1 : Outport  Port=10
  ILraw2 : Outport  Port=11
  ILraw3 : Outport  Port=12
  IRload : Outport  Port=13
  VC : Outport  Port=14
  wires:
  PS-Simulink Converter4/1 -> Gain2/1  "Vin"
  SH1/1 -> Simulink-PS Converter/1  "SH"
  PS-Simulink Converter2/1 -> Gain3/1  "Iout"
  PS-Simulink Converter1/1 -> VC/1, Gain4/1  "Vout"
  Transfer Fcn5/1 -> Vout/1  "Vout"
  PS-Simulink Converter/1 -> ILraw1/1, Gain1/1  "IL1"
  PS-Simulink Converter3/1 -> Gain7/1  "VL1"
  SL1/1 -> Simulink-PS Converter1/1  "SL"
  Transfer Fcn3/1 -> VL1/1  "VL1"
  Gain7/1 -> Transfer Fcn3/1
  Transfer Fcn1/1 -> IL1/1  "IL1"
  Transfer Fcn2/1 -> Vin/1  "Vin"
  Transfer Fcn4/1 -> Iout/1  "Iout"
  Gain1/1 -> Transfer Fcn1/1
  Gain2/1 -> Transfer Fcn2/1
  Gain3/1 -> Transfer Fcn4/1
  RloadRef/1 -> Simulink-PS Converter3/1
  SH2/1 -> Simulink-PS Converter2/1  "SH3"
  SL2/1 -> Simulink-PS Converter4/1  "SL3"
  PS-Simulink Converter7/1 -> Gain6/1  "VL2"
  Gain6/1 -> Transfer Fcn7/1
  Gain5/1 -> Transfer Fcn6/1
  Transfer Fcn7/1 -> VL2/1  "VL2"
  Transfer Fcn6/1 -> IL2/1  "IL2"
  PS-Simulink Converter6/1 -> ILraw2/1, Gain5/1  "IL2"
  SL3/1 -> Simulink-PS Converter6/1  "SL3"
  PS-Simulink Converter9/1 -> ILraw3/1, Gain9/1  "IL3"
  Transfer Fcn10/1 -> VL3/1  "VL3"
  Transfer Fcn9/1 -> IL3/1  "IL3"
  Gain9/1 -> Transfer Fcn9/1
  Gain10/1 -> Transfer Fcn10/1
  PS-Simulink Converter10/1 -> Gain10/1  "VL3"
  SH3/1 -> Simulink-PS Converter5/1  "SH3"
  Gain4/1 -> Transfer Fcn5/1
  VinRef/1 -> Simulink-PS Converter7/1  "SL"
  CB/1 -> Fcn/1
  Fcn/1 -> Simulink-PS Converter8/1
  Gain8/1 -> Transfer Fcn8/1
  PS-Simulink Converter5/1 -> Gain8/1  "Iload"
  Transfer Fcn8/1 -> IRload/1  "Iload"
  connections:
  Current Sensor/RConn1 -- PS-Simulink Converter/LConn1
  Current Sensor/RConn2 -- Voltage Sensor1/LConn1 -- Inductor/LConn1
  Voltage Sensor2/RConn2 -- Controlled Voltage Source/RConn2 -- Electrical Reference/LConn1 -- Solver Configuration1/RConn1 -- "IGBT (Ideal, Switching)1"/RConn2 -- Variable Resistor/RConn1 -- Voltage Sensor/RConn2 -- Capacitor/RConn1
  PS-Simulink Converter4/LConn1 -- Voltage Sensor2/RConn1
  Voltage Sensor2/LConn1 -- Controlled Voltage Source/LConn1 -- Connection Label2/LConn1 -- Current Sensor/LConn1
  Voltage Sensor/LConn1 -- Current Sensor3/LConn1 -- Capacitor/LConn1 -- Current Sensor1/RConn2
  Inductor/RConn1 -- Voltage Sensor1/RConn2 -- "IGBT (Ideal, Switching)1"/RConn1 -- "IGBT (Ideal, Switching)"/RConn2
  PS-Simulink Converter3/LConn1 -- Voltage Sensor1/RConn1
  "IGBT (Ideal, Switching)"/RConn1 -- Connection Label/LConn1 -- Current Sensor1/LConn1
  "IGBT (Ideal, Switching)1"/LConn1 -- Simulink-PS Converter1/RConn1
  PS-Simulink Converter2/LConn1 -- Current Sensor1/RConn1
  PS-Simulink Converter1/LConn1 -- Voltage Sensor/RConn1
  Simulink-PS Converter/RConn1 -- "IGBT (Ideal, Switching)"/LConn1
  Variable Resistor/LConn1 -- Simulink-PS Converter3/RConn1
  "IGBT (Ideal, Switching)2"/RConn2 -- Inductor1/RConn1 -- Voltage Sensor3/RConn2 -- "IGBT (Ideal, Switching)3"/RConn1
  Inductor1/LConn1 -- Current Sensor2/RConn2 -- Voltage Sensor3/LConn1
  "IGBT (Ideal, Switching)3"/RConn2 -- Electrical Reference1/LConn1
  "IGBT (Ideal, Switching)3"/LConn1 -- Simulink-PS Converter4/RConn1
  Simulink-PS Converter2/RConn1 -- "IGBT (Ideal, Switching)2"/LConn1
  Connection Label3/LConn1 -- Current Sensor2/LConn1
  PS-Simulink Converter7/LConn1 -- Voltage Sensor3/RConn1
  PS-Simulink Converter6/LConn1 -- Current Sensor2/RConn1
  "IGBT (Ideal, Switching)4"/RConn2 -- "IGBT (Ideal, Switching)5"/RConn1 -- Inductor2/RConn1 -- Voltage Sensor4/RConn2
  Inductor2/LConn1 -- Current Sensor4/RConn2 -- Voltage Sensor4/LConn1
  "IGBT (Ideal, Switching)5"/LConn1 -- Simulink-PS Converter6/RConn1
  PS-Simulink Converter10/LConn1 -- Voltage Sensor4/RConn1
  Simulink-PS Converter5/RConn1 -- "IGBT (Ideal, Switching)4"/LConn1
  "IGBT (Ideal, Switching)5"/RConn2 -- Electrical Reference2/LConn1
  PS-Simulink Converter9/LConn1 -- Current Sensor4/RConn1
  Connection Label5/LConn1 -- Current Sensor4/LConn1
  Connection Label1/LConn1 -- "IGBT (Ideal, Switching)2"/RConn1
  Connection Label4/LConn1 -- "IGBT (Ideal, Switching)4"/RConn1
  Simulink-PS Converter7/RConn1 -- Controlled Voltage Source/RConn1
  Circuit Breaker/LConn2 -- Variable Resistor/LConn2
  Simulink-PS Converter8/RConn1 -- Circuit Breaker/LConn1
  Current Sensor3/RConn2 -- Circuit Breaker/RConn1
  PS-Simulink Converter5/LConn1 -- Current Sensor3/RConn1

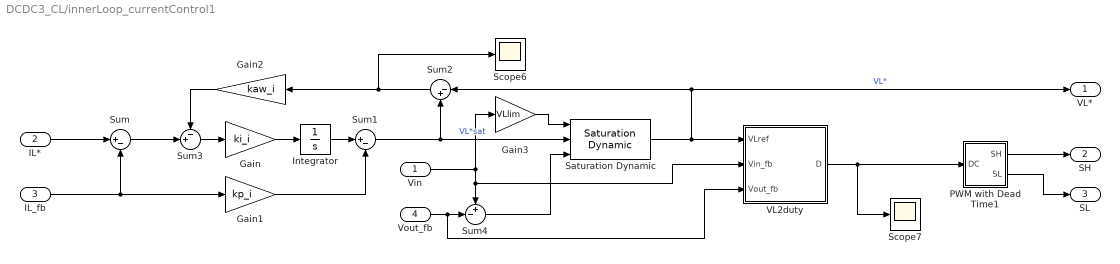
== system DCDC3_CL/innerLoop_currentControl1 ==
  Vin : Inport
  IL* : Inport  Port=2
  IL_fb : Inport  Port=3
  Vout_fb : Inport  Port=4
  Gain : Gain  Gain=ki_i
  Gain1 : Gain  Gain=kp_i
  Gain2 : Gain  Gain=kaw_i
  Gain3 : Gain  Gain=VLlim
  Integrator : Integrator
  PWM with Dead Time1 : Subsystem
  Saturation Dynamic : simulink/Discontinuities/Saturation Dynamic  OutMin=[]  OutMax=[]  OutDataTypeStr=Inherit: Same as second input  OutDataType=fixdt(1, 16)  OutScaling=2^-10  DoSatur=off
  Scope6 : Scope
  Scope7 : Scope
  Sum : Sum  Inputs=|+-
  Sum1 : Sum  Inputs=|+-
  Sum2 : Sum  Inputs=|-+
  Sum3 : Sum  Inputs=-+|
  Sum4 : Sum  Inputs=+-|
  VL2duty : MATLAB Function  TreatAsAtomicUnit=on
  VL* : Outport
  SH : Outport  Port=2
  SL : Outport  Port=3
  wires:
  VL2duty/1(D) -> PWM with Dead Time1/1(DC), Scope7/1
  Sum/1 -> Sum3/2
  Gain3/1 -> Saturation Dynamic/1
  Gain1/1 -> Sum1/2
  Sum3/1 -> Gain/1
  Gain/1 -> Integrator/1
  Gain2/1 -> Sum3/1
  PWM with Dead Time1/2(SL) -> SL/1
  Vin/1 -> VL2duty/2(Vin_fb), Sum4/1, Gain3/1
  Sum1/1 -> Saturation Dynamic/2, Sum2/2  "VL*sat"
  Sum4/1 -> Saturation Dynamic/3
  Sum2/1 -> Gain2/1, Scope6/1
  Saturation Dynamic/1 -> VL2duty/1(VLref), VL*/1, Sum2/1  "VL*"
  IL_fb/1 -> Sum/2, Gain1/1
  Vout_fb/1 -> VL2duty/3(Vout_fb), Sum4/2
  Integrator/1 -> Sum1/1
  PWM with Dead Time1/1(SH) -> SH/1
  IL*/1 -> Sum/1

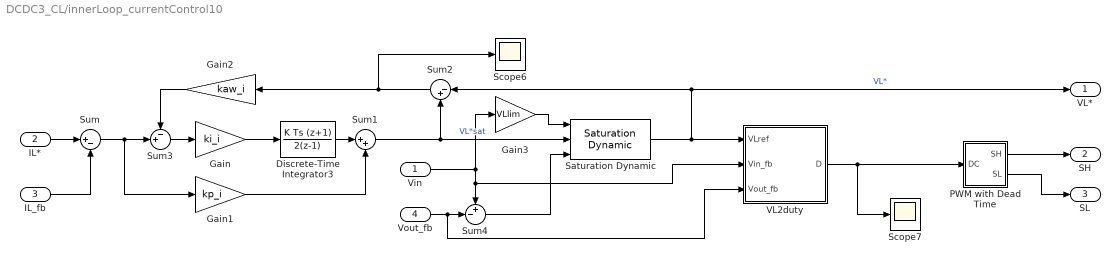
== system DCDC3_CL/innerLoop_currentControl10 ==
  Vin : Inport
  IL* : Inport  Port=2
  IL_fb : Inport  Port=3
  Vout_fb : Inport  Port=4
  Discrete-Time Integrator3 : DiscreteIntegrator  IntegratorMethod=Integration: Trapezoidal  SampleTime=Tsw  ICPrevOutput=DiscIntNeverNeededParam  ICPrevScaledInput=DiscIntNeverNeededParam
  Gain : Gain  Gain=ki_i
  Gain1 : Gain  Gain=kp_i
  Gain2 : Gain  Gain=kaw_i
  Gain3 : Gain  Gain=VLlim
  PWM with Dead Time : Subsystem
  Saturation Dynamic : simulink/Discontinuities/Saturation Dynamic  OutMin=[]  OutMax=[]  OutDataTypeStr=Inherit: Same as second input  OutDataType=fixdt(1, 16)  OutScaling=2^-10  DoSatur=off
  Scope6 : Scope
  Scope7 : Scope
  Sum : Sum  Inputs=|+-
  Sum1 : Sum  Inputs=|++
  Sum2 : Sum  Inputs=|-+
  Sum3 : Sum  Inputs=-+|
  Sum4 : Sum  Inputs=+-|
  VL2duty : MATLAB Function  TreatAsAtomicUnit=on
  VL* : Outport
  SH : Outport  Port=2
  SL : Outport  Port=3
  wires:
  VL2duty/1(D) -> PWM with Dead Time/1(DC), Scope7/1
  Sum/1 -> Gain1/1, Sum3/2
  Gain3/1 -> Saturation Dynamic/1
  Gain1/1 -> Sum1/2
  Sum3/1 -> Gain/1
  Gain/1 -> Discrete-Time Integrator3/1
  Gain2/1 -> Sum3/1
  PWM with Dead Time/2(SL) -> SL/1
  Vin/1 -> VL2duty/2(Vin_fb), Sum4/1, Gain3/1
  Sum1/1 -> Saturation Dynamic/2, Sum2/2  "VL*sat"
  Sum4/1 -> Saturation Dynamic/3
  Sum2/1 -> Gain2/1, Scope6/1
  Saturation Dynamic/1 -> VL2duty/1(VLref), VL*/1, Sum2/1  "VL*"
  IL_fb/1 -> Sum/2
  Vout_fb/1 -> VL2duty/3(Vout_fb), Sum4/2
  Discrete-Time Integrator3/1 -> Sum1/1
  PWM with Dead Time/1(SH) -> SH/1
  IL*/1 -> Sum/1

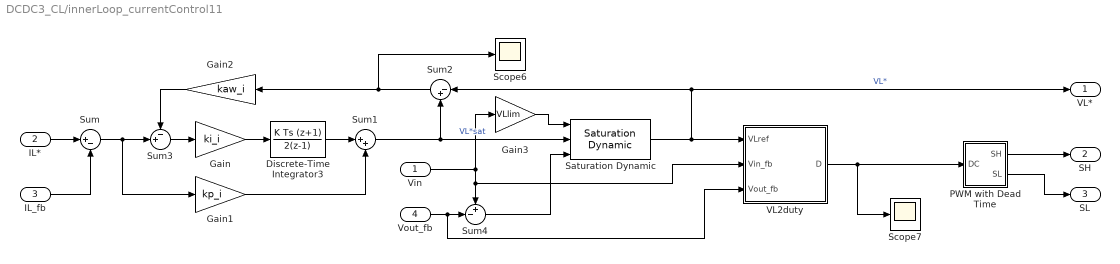
== system DCDC3_CL/innerLoop_currentControl11 ==
  Vin : Inport
  IL* : Inport  Port=2
  IL_fb : Inport  Port=3
  Vout_fb : Inport  Port=4
  Discrete-Time Integrator3 : DiscreteIntegrator  IntegratorMethod=Integration: Trapezoidal  SampleTime=Tsw  ICPrevOutput=DiscIntNeverNeededParam  ICPrevScaledInput=DiscIntNeverNeededParam
  Gain : Gain  Gain=ki_i
  Gain1 : Gain  Gain=kp_i
  Gain2 : Gain  Gain=kaw_i
  Gain3 : Gain  Gain=VLlim
  PWM with Dead Time : Subsystem
  Saturation Dynamic : simulink/Discontinuities/Saturation Dynamic  OutMin=[]  OutMax=[]  OutDataTypeStr=Inherit: Same as second input  OutDataType=fixdt(1, 16)  OutScaling=2^-10  DoSatur=off
  Scope6 : Scope
  Scope7 : Scope
  Sum : Sum  Inputs=|+-
  Sum1 : Sum  Inputs=|++
  Sum2 : Sum  Inputs=|-+
  Sum3 : Sum  Inputs=-+|
  Sum4 : Sum  Inputs=+-|
  VL2duty : MATLAB Function  TreatAsAtomicUnit=on
  VL* : Outport
  SH : Outport  Port=2
  SL : Outport  Port=3
  wires:
  Sum/1 -> Gain1/1, Sum3/2
  Gain3/1 -> Saturation Dynamic/1
  Gain1/1 -> Sum1/2
  Sum3/1 -> Gain/1
  Gain/1 -> Discrete-Time Integrator3/1
  Gain2/1 -> Sum3/1
  PWM with Dead Time/2(SL) -> SL/1
  Vin/1 -> VL2duty/2(Vin_fb), Sum4/1, Gain3/1
  Sum1/1 -> Saturation Dynamic/2, Sum2/2  "VL*sat"
  Sum4/1 -> Saturation Dynamic/3
  Sum2/1 -> Gain2/1, Scope6/1
  Saturation Dynamic/1 -> VL2duty/1(VLref), VL*/1, Sum2/1  "VL*"
  Vout_fb/1 -> VL2duty/3(Vout_fb), Sum4/2
  Discrete-Time Integrator3/1 -> Sum1/1
  PWM with Dead Time/1(SH) -> SH/1
  IL*/1 -> Sum/1
  VL2duty/1(D) -> PWM with Dead Time/1(DC), Scope7/1
  IL_fb/1 -> Sum/2

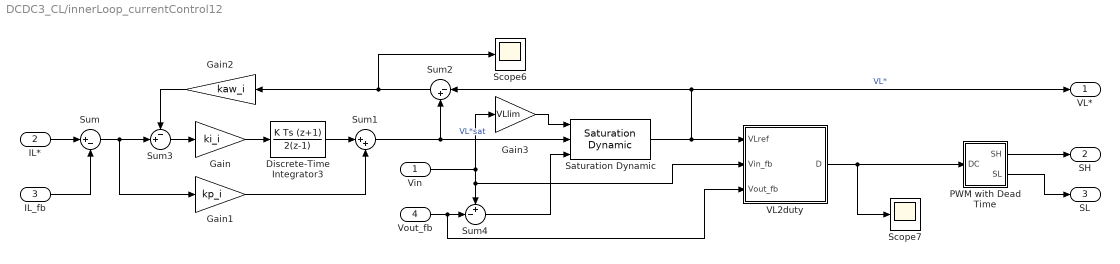
== system DCDC3_CL/innerLoop_currentControl12 ==
  Vin : Inport
  IL* : Inport  Port=2
  IL_fb : Inport  Port=3
  Vout_fb : Inport  Port=4
  Discrete-Time Integrator3 : DiscreteIntegrator  IntegratorMethod=Integration: Trapezoidal  SampleTime=Tsw  ICPrevOutput=DiscIntNeverNeededParam  ICPrevScaledInput=DiscIntNeverNeededParam
  Gain : Gain  Gain=ki_i
  Gain1 : Gain  Gain=kp_i
  Gain2 : Gain  Gain=kaw_i
  Gain3 : Gain  Gain=VLlim
  PWM with Dead Time : Subsystem
  Saturation Dynamic : simulink/Discontinuities/Saturation Dynamic  OutMin=[]  OutMax=[]  OutDataTypeStr=Inherit: Same as second input  OutDataType=fixdt(1, 16)  OutScaling=2^-10  DoSatur=off
  Scope6 : Scope
  Scope7 : Scope
  Sum : Sum  Inputs=|+-
  Sum1 : Sum  Inputs=|++
  Sum2 : Sum  Inputs=|-+
  Sum3 : Sum  Inputs=-+|
  Sum4 : Sum  Inputs=+-|
  VL2duty : MATLAB Function  TreatAsAtomicUnit=on
  VL* : Outport
  SH : Outport  Port=2
  SL : Outport  Port=3
  wires:
  Sum/1 -> Gain1/1, Sum3/2
  Gain3/1 -> Saturation Dynamic/1
  Gain1/1 -> Sum1/2
  Sum3/1 -> Gain/1
  Gain/1 -> Discrete-Time Integrator3/1
  Gain2/1 -> Sum3/1
  PWM with Dead Time/2(SL) -> SL/1
  Vin/1 -> VL2duty/2(Vin_fb), Sum4/1, Gain3/1
  Sum1/1 -> Saturation Dynamic/2, Sum2/2  "VL*sat"
  Sum4/1 -> Saturation Dynamic/3
  Sum2/1 -> Gain2/1, Scope6/1
  Saturation Dynamic/1 -> VL2duty/1(VLref), VL*/1, Sum2/1  "VL*"
  IL_fb/1 -> Sum/2
  Vout_fb/1 -> VL2duty/3(Vout_fb), Sum4/2
  Discrete-Time Integrator3/1 -> Sum1/1
  PWM with Dead Time/1(SH) -> SH/1
  IL*/1 -> Sum/1
  VL2duty/1(D) -> PWM with Dead Time/1(DC), Scope7/1

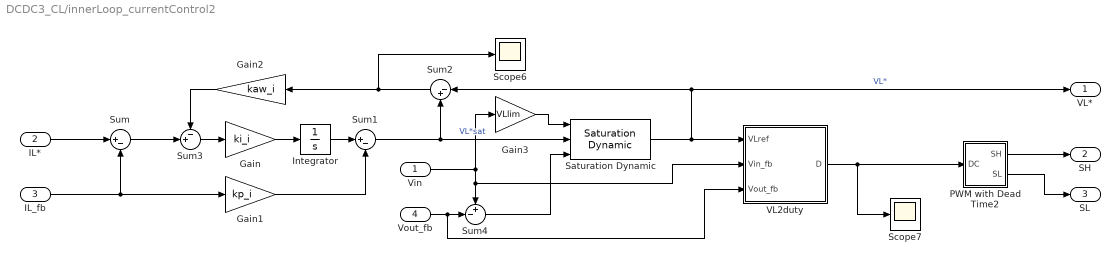
== system DCDC3_CL/innerLoop_currentControl2 ==
  Vin : Inport
  IL* : Inport  Port=2
  IL_fb : Inport  Port=3
  Vout_fb : Inport  Port=4
  Gain : Gain  Gain=ki_i
  Gain1 : Gain  Gain=kp_i
  Gain2 : Gain  Gain=kaw_i
  Gain3 : Gain  Gain=VLlim
  Integrator : Integrator
  PWM with Dead Time2 : Subsystem
  Saturation Dynamic : simulink/Discontinuities/Saturation Dynamic  OutMin=[]  OutMax=[]  OutDataTypeStr=Inherit: Same as second input  OutDataType=fixdt(1, 16)  OutScaling=2^-10  DoSatur=off
  Scope6 : Scope
  Scope7 : Scope
  Sum : Sum  Inputs=|+-
  Sum1 : Sum  Inputs=|+-
  Sum2 : Sum  Inputs=|-+
  Sum3 : Sum  Inputs=-+|
  Sum4 : Sum  Inputs=+-|
  VL2duty : MATLAB Function  TreatAsAtomicUnit=on
  VL* : Outport
  SH : Outport  Port=2
  SL : Outport  Port=3
  wires:
  Sum/1 -> Sum3/2
  Gain3/1 -> Saturation Dynamic/1
  Gain1/1 -> Sum1/2
  Sum3/1 -> Gain/1
  Gain/1 -> Integrator/1
  Gain2/1 -> Sum3/1
  PWM with Dead Time2/2(SL) -> SL/1
  Vin/1 -> VL2duty/2(Vin_fb), Sum4/1, Gain3/1
  Sum1/1 -> Saturation Dynamic/2, Sum2/2  "VL*sat"
  Sum4/1 -> Saturation Dynamic/3
  Sum2/1 -> Gain2/1, Scope6/1
  Saturation Dynamic/1 -> VL2duty/1(VLref), VL*/1, Sum2/1  "VL*"
  Vout_fb/1 -> VL2duty/3(Vout_fb), Sum4/2
  Integrator/1 -> Sum1/1
  PWM with Dead Time2/1(SH) -> SH/1
  IL*/1 -> Sum/1
  VL2duty/1(D) -> PWM with Dead Time2/1(DC), Scope7/1
  IL_fb/1 -> Sum/2, Gain1/1

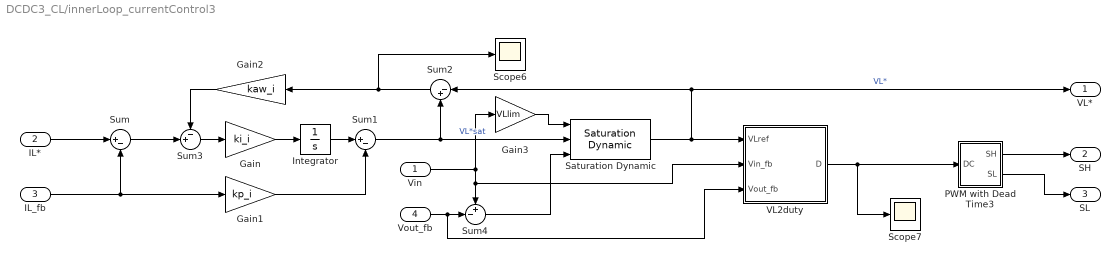
== system DCDC3_CL/innerLoop_currentControl3 ==
  Vin : Inport
  IL* : Inport  Port=2
  IL_fb : Inport  Port=3
  Vout_fb : Inport  Port=4
  Gain : Gain  Gain=ki_i
  Gain1 : Gain  Gain=kp_i
  Gain2 : Gain  Gain=kaw_i
  Gain3 : Gain  Gain=VLlim
  Integrator : Integrator
  PWM with Dead Time3 : Subsystem
  Saturation Dynamic : simulink/Discontinuities/Saturation Dynamic  OutMin=[]  OutMax=[]  OutDataTypeStr=Inherit: Same as second input  OutDataType=fixdt(1, 16)  OutScaling=2^-10  DoSatur=off
  Scope6 : Scope
  Scope7 : Scope
  Sum : Sum  Inputs=|+-
  Sum1 : Sum  Inputs=|+-
  Sum2 : Sum  Inputs=|-+
  Sum3 : Sum  Inputs=-+|
  Sum4 : Sum  Inputs=+-|
  VL2duty : MATLAB Function  TreatAsAtomicUnit=on
  VL* : Outport
  SH : Outport  Port=2
  SL : Outport  Port=3
  wires:
  Sum/1 -> Sum3/2
  Gain3/1 -> Saturation Dynamic/1
  Gain1/1 -> Sum1/2
  Sum3/1 -> Gain/1
  Gain/1 -> Integrator/1
  Gain2/1 -> Sum3/1
  PWM with Dead Time3/2(SL) -> SL/1
  Vin/1 -> VL2duty/2(Vin_fb), Sum4/1, Gain3/1
  Sum1/1 -> Saturation Dynamic/2, Sum2/2  "VL*sat"
  Sum4/1 -> Saturation Dynamic/3
  Sum2/1 -> Gain2/1, Scope6/1
  Saturation Dynamic/1 -> VL2duty/1(VLref), VL*/1, Sum2/1  "VL*"
  IL_fb/1 -> Sum/2, Gain1/1
  Vout_fb/1 -> VL2duty/3(Vout_fb), Sum4/2
  Integrator/1 -> Sum1/1
  PWM with Dead Time3/1(SH) -> SH/1
  IL*/1 -> Sum/1
  VL2duty/1(D) -> PWM with Dead Time3/1(DC), Scope7/1

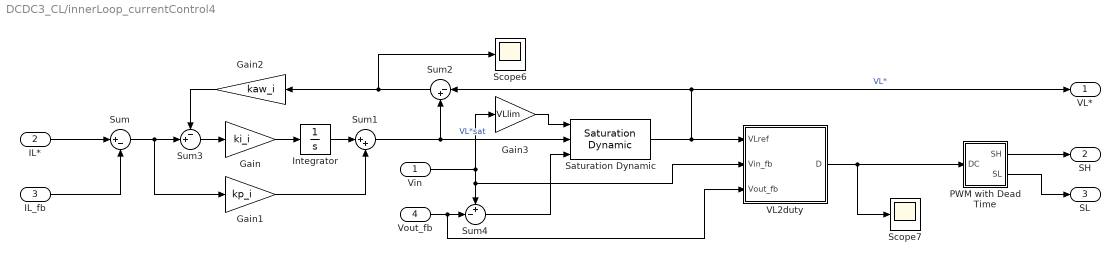
== system DCDC3_CL/innerLoop_currentControl4 ==
  Vin : Inport
  IL* : Inport  Port=2
  IL_fb : Inport  Port=3
  Vout_fb : Inport  Port=4
  Gain : Gain  Gain=ki_i
  Gain1 : Gain  Gain=kp_i
  Gain2 : Gain  Gain=kaw_i
  Gain3 : Gain  Gain=VLlim
  Integrator : Integrator
  PWM with Dead Time : Subsystem
  Saturation Dynamic : simulink/Discontinuities/Saturation Dynamic  OutMin=[]  OutMax=[]  OutDataTypeStr=Inherit: Same as second input  OutDataType=fixdt(1, 16)  OutScaling=2^-10  DoSatur=off
  Scope6 : Scope
  Scope7 : Scope
  Sum : Sum  Inputs=|+-
  Sum1 : Sum  Inputs=|++
  Sum2 : Sum  Inputs=|-+
  Sum3 : Sum  Inputs=-+|
  Sum4 : Sum  Inputs=+-|
  VL2duty : MATLAB Function  TreatAsAtomicUnit=on
  VL* : Outport
  SH : Outport  Port=2
  SL : Outport  Port=3
  wires:
  VL2duty/1(D) -> PWM with Dead Time/1(DC), Scope7/1
  Sum/1 -> Gain1/1, Sum3/2
  Gain3/1 -> Saturation Dynamic/1
  Gain1/1 -> Sum1/2
  Sum3/1 -> Gain/1
  Gain/1 -> Integrator/1
  Gain2/1 -> Sum3/1
  PWM with Dead Time/2(SL) -> SL/1
  Vin/1 -> VL2duty/2(Vin_fb), Sum4/1, Gain3/1
  Sum1/1 -> Saturation Dynamic/2, Sum2/2  "VL*sat"
  Sum4/1 -> Saturation Dynamic/3
  Sum2/1 -> Gain2/1, Scope6/1
  Saturation Dynamic/1 -> VL2duty/1(VLref), VL*/1, Sum2/1  "VL*"
  IL_fb/1 -> Sum/2
  Vout_fb/1 -> VL2duty/3(Vout_fb), Sum4/2
  Integrator/1 -> Sum1/1
  PWM with Dead Time/1(SH) -> SH/1
  IL*/1 -> Sum/1

== system DCDC3_CL/innerLoop_currentControl5 ==
  Vin : Inport
  IL* : Inport  Port=2
  IL_fb : Inport  Port=3
  Vout_fb : Inport  Port=4
  Gain : Gain  Gain=ki_i
  Gain1 : Gain  Gain=kp_i
  Gain2 : Gain  Gain=kaw_i
  Gain3 : Gain  Gain=VLlim
  Integrator : Integrator
  PWM with Dead Time : Subsystem
  Saturation Dynamic : simulink/Discontinuities/Saturation Dynamic  OutMin=[]  OutMax=[]  OutDataTypeStr=Inherit: Same as second input  OutDataType=fixdt(1, 16)  OutScaling=2^-10  DoSatur=off
  Scope6 : Scope
  Scope7 : Scope
  Sum : Sum  Inputs=|+-
  Sum1 : Sum  Inputs=|++
  Sum2 : Sum  Inputs=|-+
  Sum3 : Sum  Inputs=-+|
  Sum4 : Sum  Inputs=+-|
  VL2duty : MATLAB Function  TreatAsAtomicUnit=on
  VL* : Outport
  SH : Outport  Port=2
  SL : Outport  Port=3
  wires:
  Sum/1 -> Gain1/1, Sum3/2
  Gain3/1 -> Saturation Dynamic/1
  Gain1/1 -> Sum1/2
  Sum3/1 -> Gain/1
  Gain/1 -> Integrator/1
  Gain2/1 -> Sum3/1
  PWM with Dead Time/2(SL) -> SL/1
  Vin/1 -> VL2duty/2(Vin_fb), Sum4/1, Gain3/1
  Sum1/1 -> Saturation Dynamic/2, Sum2/2  "VL*sat"
  Sum4/1 -> Saturation Dynamic/3
  Sum2/1 -> Gain2/1, Scope6/1
  Saturation Dynamic/1 -> VL2duty/1(VLref), VL*/1, Sum2/1  "VL*"
  Vout_fb/1 -> VL2duty/3(Vout_fb), Sum4/2
  Integrator/1 -> Sum1/1
  PWM with Dead Time/1(SH) -> SH/1
  IL*/1 -> Sum/1
  VL2duty/1(D) -> PWM with Dead Time/1(DC), Scope7/1
  IL_fb/1 -> Sum/2

== system DCDC3_CL/innerLoop_currentControl6 ==
  Vin : Inport
  IL* : Inport  Port=2
  IL_fb : Inport  Port=3
  Vout_fb : Inport  Port=4
  Gain : Gain  Gain=ki_i
  Gain1 : Gain  Gain=kp_i
  Gain2 : Gain  Gain=kaw_i
  Gain3 : Gain  Gain=VLlim
  Integrator : Integrator
  PWM with Dead Time : Subsystem
  Saturation Dynamic : simulink/Discontinuities/Saturation Dynamic  OutMin=[]  OutMax=[]  OutDataTypeStr=Inherit: Same as second input  OutDataType=fixdt(1, 16)  OutScaling=2^-10  DoSatur=off
  Scope6 : Scope
  Scope7 : Scope
  Sum : Sum  Inputs=|+-
  Sum1 : Sum  Inputs=|++
  Sum2 : Sum  Inputs=|-+
  Sum3 : Sum  Inputs=-+|
  Sum4 : Sum  Inputs=+-|
  VL2duty : MATLAB Function  TreatAsAtomicUnit=on
  VL* : Outport
  SH : Outport  Port=2
  SL : Outport  Port=3
  wires:
  Sum/1 -> Gain1/1, Sum3/2
  Gain3/1 -> Saturation Dynamic/1
  Gain1/1 -> Sum1/2
  Sum3/1 -> Gain/1
  Gain/1 -> Integrator/1
  Gain2/1 -> Sum3/1
  PWM with Dead Time/2(SL) -> SL/1
  Vin/1 -> VL2duty/2(Vin_fb), Sum4/1, Gain3/1
  Sum1/1 -> Saturation Dynamic/2, Sum2/2  "VL*sat"
  Sum4/1 -> Saturation Dynamic/3
  Sum2/1 -> Gain2/1, Scope6/1
  Saturation Dynamic/1 -> VL2duty/1(VLref), VL*/1, Sum2/1  "VL*"
  IL_fb/1 -> Sum/2
  Vout_fb/1 -> VL2duty/3(Vout_fb), Sum4/2
  Integrator/1 -> Sum1/1
  PWM with Dead Time/1(SH) -> SH/1
  IL*/1 -> Sum/1
  VL2duty/1(D) -> PWM with Dead Time/1(DC), Scope7/1

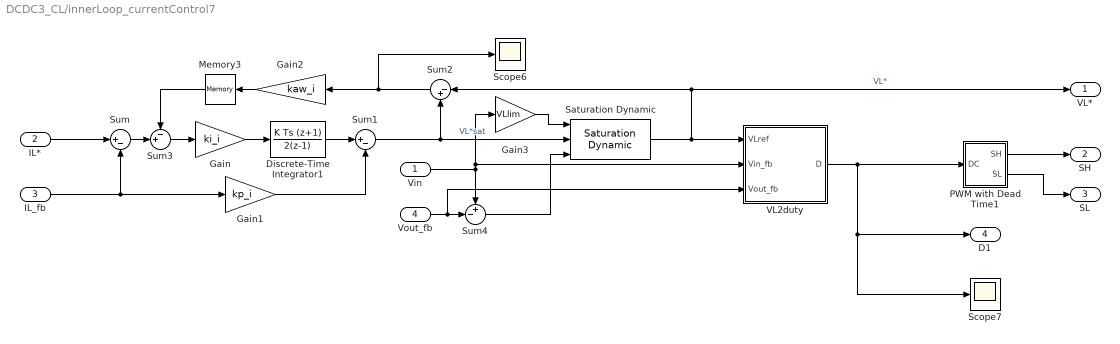
== system DCDC3_CL/innerLoop_currentControl7 ==
  Vin : Inport
  IL* : Inport  Port=2
  IL_fb : Inport  Port=3
  Vout_fb : Inport  Port=4
  Discrete-Time Integrator1 : DiscreteIntegrator  IntegratorMethod=Integration: Trapezoidal  SampleTime=Tsw  ICPrevOutput=DiscIntNeverNeededParam  ICPrevScaledInput=DiscIntNeverNeededParam
  Gain : Gain  Gain=ki_i
  Gain1 : Gain  Gain=kp_i
  Gain2 : Gain  Gain=kaw_i
  Gain3 : Gain  Gain=VLlim
  Memory3 : Memory
  PWM with Dead Time1 : Subsystem
  Saturation Dynamic : simulink/Discontinuities/Saturation Dynamic  OutMin=[]  OutMax=[]  OutDataTypeStr=Inherit: Same as second input  OutDataType=fixdt(1, 16)  OutScaling=2^-10  DoSatur=off
  Scope6 : Scope
  Scope7 : Scope
  Sum : Sum  Inputs=|+-
  Sum1 : Sum  Inputs=|+-
  Sum2 : Sum  Inputs=|-+
  Sum3 : Sum  Inputs=-+|
  Sum4 : Sum  Inputs=+-|
  VL2duty : MATLAB Function  TreatAsAtomicUnit=on
  VL* : Outport
  SH : Outport  Port=2
  SL : Outport  Port=3
  D1 : Outport  Port=4
  wires:
  VL2duty/1(D) -> PWM with Dead Time1/1(DC), Scope7/1, D1/1
  Sum/1 -> Sum3/2
  Gain3/1 -> Saturation Dynamic/1
  Gain1/1 -> Sum1/2
  Sum3/1 -> Gain/1
  Gain/1 -> Discrete-Time Integrator1/1
  Gain2/1 -> Memory3/1
  PWM with Dead Time1/2(SL) -> SL/1
  Vin/1 -> VL2duty/2(Vin_fb), Gain3/1, Sum4/1
  Sum1/1 -> Saturation Dynamic/2, Sum2/2  "VL*sat"
  Sum4/1 -> Saturation Dynamic/3
  Sum2/1 -> Gain2/1, Scope6/1
  Saturation Dynamic/1 -> VL*/1, Sum2/1, VL2duty/1(VLref)  "VL*"
  IL_fb/1 -> Sum/2, Gain1/1
  Vout_fb/1 -> VL2duty/3(Vout_fb), Sum4/2
  Discrete-Time Integrator1/1 -> Sum1/1
  PWM with Dead Time1/1(SH) -> SH/1
  IL*/1 -> Sum/1
  Memory3/1 -> Sum3/1

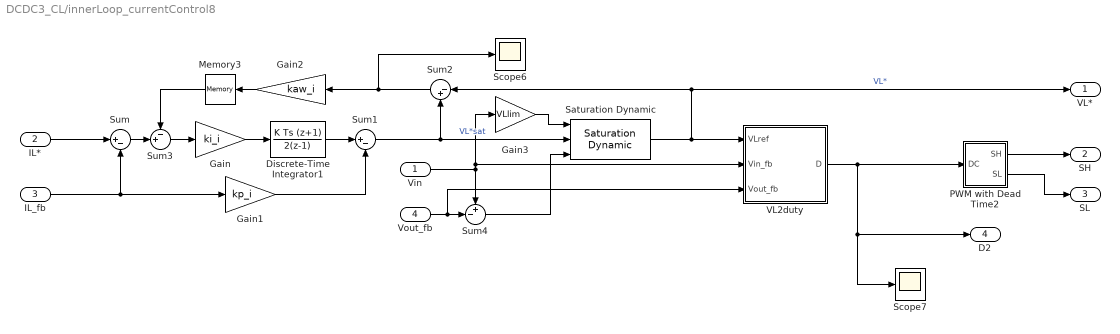
== system DCDC3_CL/innerLoop_currentControl8 ==
  Vin : Inport
  IL* : Inport  Port=2
  IL_fb : Inport  Port=3
  Vout_fb : Inport  Port=4
  Discrete-Time Integrator1 : DiscreteIntegrator  IntegratorMethod=Integration: Trapezoidal  SampleTime=Tsw  ICPrevOutput=DiscIntNeverNeededParam  ICPrevScaledInput=DiscIntNeverNeededParam
  Gain : Gain  Gain=ki_i
  Gain1 : Gain  Gain=kp_i
  Gain2 : Gain  Gain=kaw_i
  Gain3 : Gain  Gain=VLlim
  Memory3 : Memory
  PWM with Dead Time2 : Subsystem
  Saturation Dynamic : simulink/Discontinuities/Saturation Dynamic  OutMin=[]  OutMax=[]  OutDataTypeStr=Inherit: Same as second input  OutDataType=fixdt(1, 16)  OutScaling=2^-10  DoSatur=off
  Scope6 : Scope
  Scope7 : Scope
  Sum : Sum  Inputs=|+-
  Sum1 : Sum  Inputs=|+-
  Sum2 : Sum  Inputs=|-+
  Sum3 : Sum  Inputs=-+|
  Sum4 : Sum  Inputs=+-|
  VL2duty : MATLAB Function  TreatAsAtomicUnit=on
  VL* : Outport
  SH : Outport  Port=2
  SL : Outport  Port=3
  D2 : Outport  Port=4
  wires:
  Sum/1 -> Sum3/2
  Gain3/1 -> Saturation Dynamic/1
  Gain1/1 -> Sum1/2
  Sum3/1 -> Gain/1
  Gain/1 -> Discrete-Time Integrator1/1
  Gain2/1 -> Memory3/1
  PWM with Dead Time2/2(SL) -> SL/1
  Vin/1 -> VL2duty/2(Vin_fb), Gain3/1, Sum4/1
  Sum1/1 -> Saturation Dynamic/2, Sum2/2  "VL*sat"
  Sum4/1 -> Saturation Dynamic/3
  Sum2/1 -> Gain2/1, Scope6/1
  Saturation Dynamic/1 -> VL*/1, Sum2/1, VL2duty/1(VLref)  "VL*"
  Vout_fb/1 -> VL2duty/3(Vout_fb), Sum4/2
  Discrete-Time Integrator1/1 -> Sum1/1
  PWM with Dead Time2/1(SH) -> SH/1
  IL*/1 -> Sum/1
  VL2duty/1(D) -> PWM with Dead Time2/1(DC), D2/1, Scope7/1
  IL_fb/1 -> Sum/2, Gain1/1
  Memory3/1 -> Sum3/1
